simulink library "inp"  (R2021b)
settings: Solver=VariableStepAuto  StartTime=0.0  StopTime=10.0  RelTol=1e-3
undefined symbols (not defined in the file): C_TASK_5MS_S, FALSE, KINP_AcoreReadyToSlp_flg_ovrdflg, KINP_AcoreReadyToSlp_flg_ovrdval, KINP_AllowMovThd_OTA_enum_ovrdflg, KINP_AllowMovThd_OTA_enum_ovrdval, KINP_APSAngleTarget_Deg_ovrdflg, KINP_APSAngleTarget_Deg_ovrdval, KINP_APSDecReq_mps2_ovrdflg, KINP_APSDecReq_mps2_ovrdval, KINP_APSDecReqA_flg_ovrdflg, KINP_APSDecReqA_flg_ovrdval, KINP_APSDFLL_cm_ovrdflg, KINP_APSDFLL_cm_ovrdval, KINP_APSDFLR_cm_ovrdflg, KINP_APSDFLR_cm_ovrdval, KINP_APSDRLL_cm_ovrdflg, KINP_APSDRLL_cm_ovrdval, KINP_APSDRLR_cm_ovrdflg, KINP_APSDRLR_cm_ovrdval, KINP_APSExitCondition_enum_ovrdflg, KINP_APSExitCondition_enum_ovrdval, KINP_APSHWVer_enum_ovrdflg, KINP_APSHWVer_enum_ovrdval, KINP_APSProgressPCT_pct_ovrdflg, KINP_APSProgressPCT_pct_ovrdval, KINP_APSPwrReq_enum_ovrdflg, KINP_APSPwrReq_enum_ovrdval, KINP_APSReq_enum_ovrdflg, KINP_APSReq_enum_ovrdval, KINP_APSRQDisplay_enum_ovrdflg, KINP_APSRQDisplay_enum_ovrdval, KINP_APSRqEPASCtrl_flg_ovrdflg, KINP_APSRqEPASCtrl_flg_ovrdval, KINP_APSShiftPosnReq_enum_ovrdval, KINP_APSShiftPosnReq_enum_ovrflg, KINP_APSSpeedCMD_kph_ovrdval, KINP_APSSpeedCMD_kph_ovrflg, KINP_APSStaSystem_enum_ovrdflg, KINP_APSStaSystem_enum_ovrdval, KINP_APSSWVer_enum_ovrdflg, KINP_APSSWVer_enum_ovrdval, KINP_APSVMCReqA_flg_ovrdval, KINP_APSVMCReqA_flg_ovrflg, KINP_APSVRqEPASCtrl_flg_ovrdflg, KINP_APSVRqEPASCtrl_flg_ovrdval, KINP_AuxBattVolmV_mV_ovrdflg, KINP_AuxBattVolmV_mV_ovrdval, KINP_BTConnectSta_enum_ovrdflg, KINP_BTConnectSta_enum_ovrdval, KINP_CAASSta_enum_ovrdflg, KINP_CAASSta_enum_ovrdval, KINP_CAASVMCReqA_flg_ovrdval, KINP_CAASVMCReqA_flg_ovrflg, KINP_CAN1BusOff_flg_ovrdflg, KINP_CAN1BusOff_flg_ovrdval, KINP_CAN2BusOff_flg_ovrdflg, KINP_CAN2BusOff_flg_ovrdval, KINP_CAN3BusOff_flg_ovrdflg, KINP_CAN3BusOff_flg_ovrdval ... (+222)
libraries: FVT_lib x1035, hcu_lib x1
(part 21 of 33)

== system inp/INP/CAN3/SignalCheck/CCU2 ==
  BHAL_outputs : Inport
  inp_CanValid_bus : Inport  Port=2
  CCU2CSErr : FVT_lib/inp/can_signal_template  SystemSampleTime=-1  VariantActivationTime=update diagram  Latency=0  AutoFrameSizeCalculation=off
      link override defval: Value=KINP_CCU2CSErr_flg_defval
      link override ovrdflg: Value=KINP_CCU2CSErr_flg_ovrdflg
      link override ovrdval: Value=KINP_CCU2CSErr_flg_ovrdval
  CCU2RCErr : FVT_lib/inp/can_signal_template  SystemSampleTime=-1  VariantActivationTime=update diagram  Latency=0  AutoFrameSizeCalculation=off
      link override defval: Value=KINP_CCU2RCErr_flg_defval
      link override ovrdflg: Value=KINP_CCU2RCErr_flg_ovrdflg
      link override ovrdval: Value=KINP_CCU2RCErr_flg_ovrdval
  CSCCU2 : FVT_lib/inp/can_signal_template  SystemSampleTime=-1  VariantActivationTime=update diagram  Latency=0  AutoFrameSizeCalculation=off
      link override defval: Value=KINP_CSCCU2_enum_defval
      link override ovrdflg: Value=KINP_CSCCU2_enum_ovrdflg
      link override ovrdval: Value=KINP_CSCCU2_enum_ovrdval
  DCDCEnaSta : FVT_lib/inp/can_signal_template  SystemSampleTime=-1  VariantActivationTime=update diagram  Latency=0  AutoFrameSizeCalculation=off
      link override defval: Value=KINP_DCDCEnaSta_flg_defval
      link override ovrdflg: Value=KINP_DCDCEnaSta_flg_ovrdflg
      link override ovrdval: Value=KINP_DCDCEnaSta_flg_ovrdval
  DCDCFaultSta : FVT_lib/inp/can_signal_template  SystemSampleTime=-1  VariantActivationTime=update diagram  Latency=0  AutoFrameSizeCalculation=off
      link override defval: Value=KINP_DCDCFaultSta_enum_defval
      link override ovrdflg: Value=KINP_DCDCFaultSta_enum_ovrdflg
      link override ovrdval: Value=KINP_DCDCFaultSta_enum_ovrdval
  DCDCReady4Pre : FVT_lib/inp/can_signal_template  SystemSampleTime=-1  VariantActivationTime=update diagram  Latency=0  AutoFrameSizeCalculation=off
      link override defval: Value=KINP_DCDCReady4Pre_flg_defval
      link override ovrdflg: Value=KINP_DCDCReady4Pre_flg_ovrdflg
      link override ovrdval: Value=KINP_DCDCReady4Pre_flg_ovrdval
  DCDCTemp : FVT_lib/inp/can_signal_template  SystemSampleTime=-1  VariantActivationTime=update diagram  Latency=0  AutoFrameSizeCalculation=off
      link override defval: Value=KINP_DCDCTemp_C_defval
      link override ovrdflg: Value=KINP_DCDCTemp_C_ovrdflg
      link override ovrdval: Value=KINP_DCDCTemp_C_ovrdval
  OBCACCurLim : FVT_lib/inp/can_signal_template  SystemSampleTime=-1  VariantActivationTime=update diagram  Latency=0  AutoFrameSizeCalculation=off
      link override defval: Value=KINP_OBCACCurLim_enum_defval
      link override ovrdflg: Value=KINP_OBCACCurLim_enum_ovrdflg
      link override ovrdval: Value=KINP_OBCACCurLim_enum_ovrdval
  OBCACCurrInf : FVT_lib/inp/can_signal_template  SystemSampleTime=-1  VariantActivationTime=update diagram  Latency=0  AutoFrameSizeCalculation=off
      link override defval: Value=KINP_OBCACCurrInf_A_defval
      link override ovrdflg: Value=KINP_OBCACCurrInf_A_ovrdflg
      link override ovrdval: Value=KINP_OBCACCurrInf_A_ovrdval
  OBCACVoltInf : FVT_lib/inp/can_signal_template  SystemSampleTime=-1  VariantActivationTime=update diagram  Latency=0  AutoFrameSizeCalculation=off
      link override defval: Value=KINP_OBCACVoltInf_V_defval
      link override ovrdflg: Value=KINP_OBCACVoltInf_V_ovrdflg
      link override ovrdval: Value=KINP_OBCACVoltInf_V_ovrdval
  OBCEnaSta : FVT_lib/inp/can_signal_template  SystemSampleTime=-1  VariantActivationTime=update diagram  Latency=0  AutoFrameSizeCalculation=off
      link override defval: Value=KINP_OBCEnaSta_flg_defval
      link override ovrdflg: Value=KINP_OBCEnaSta_flg_ovrdflg
      link override ovrdval: Value=KINP_OBCEnaSta_flg_ovrdval
  OBCFaultSta : FVT_lib/inp/can_signal_template  SystemSampleTime=-1  VariantActivationTime=update diagram  Latency=0  AutoFrameSizeCalculation=off
      link override defval: Value=KINP_OBCFaultSta_enum_defval
      link override ovrdflg: Value=KINP_OBCFaultSta_enum_ovrdflg
      link override ovrdval: Value=KINP_OBCFaultSta_enum_ovrdval
  OBCPluginSta : FVT_lib/inp/can_signal_template  SystemSampleTime=-1  VariantActivationTime=update diagram  Latency=0  AutoFrameSizeCalculation=off
      link override defval: Value=KINP_OBCPluginSta_flg_defval
      link override ovrdflg: Value=KINP_OBCPluginSta_flg_ovrdflg
      link override ovrdval: Value=KINP_OBCPluginSta_flg_ovrdval
  OBCReady4Pre : FVT_lib/inp/can_signal_template  SystemSampleTime=-1  VariantActivationTime=update diagram  Latency=0  AutoFrameSizeCalculation=off
      link override defval: Value=KINP_OBCReady4Pre_flg_defval
      link override ovrdflg: Value=KINP_OBCReady4Pre_flg_ovrdflg
      link override ovrdval: Value=KINP_OBCReady4Pre_flg_ovrdval
  OBCTemp : FVT_lib/inp/can_signal_template  SystemSampleTime=-1  VariantActivationTime=update diagram  Latency=0  AutoFrameSizeCalculation=off
      link override defval: Value=KINP_OBCTemp_C_defval
      link override ovrdflg: Value=KINP_OBCTemp_C_ovrdflg
      link override ovrdval: Value=KINP_OBCTemp_C_ovrdval
  OBCV2LSta : FVT_lib/inp/can_signal_template  SystemSampleTime=-1  VariantActivationTime=update diagram  Latency=0  AutoFrameSizeCalculation=off
      link override defval: Value=KINP_OBCV2LSta_enum_defval
      link override ovrdflg: Value=KINP_OBCV2LSta_enum_ovrdflg
      link override ovrdval: Value=KINP_OBCV2LSta_enum_ovrdval
  RCCCU2 : FVT_lib/inp/can_signal_template  SystemSampleTime=-1  VariantActivationTime=update diagram  Latency=0  AutoFrameSizeCalculation=off
      link override defval: Value=KINP_RCCCU2_enum_defval
      link override ovrdflg: Value=KINP_RCCCU2_enum_ovrdflg
      link override ovrdval: Value=KINP_RCCCU2_enum_ovrdval
  Terminator_{1..17} (17 alike) : Terminator
  True_VHAL_CCU2CSErr_flg : Constant  Value=TRUE  OutDataTypeStr=boolean
  True_VHAL_CCU2RCErr_flg : Constant  Value=TRUE  OutDataTypeStr=boolean
  True_VHAL_CSCCU2_enum : Constant  Value=TRUE  OutDataTypeStr=boolean
  True_VHAL_DCDCEnaSta_flg : Constant  Value=TRUE  OutDataTypeStr=boolean
  True_VHAL_DCDCFaultSta_enum : Constant  Value=TRUE  OutDataTypeStr=boolean
  True_VHAL_DCDCReady4Pre_flg : Constant  Value=TRUE  OutDataTypeStr=boolean
  True_VHAL_DCDCTemp_C : Constant  Value=TRUE  OutDataTypeStr=boolean
  True_VHAL_OBCACCurLim_enum : Constant  Value=TRUE  OutDataTypeStr=boolean
  True_VHAL_OBCACCurrInf_A : Constant  Value=TRUE  OutDataTypeStr=boolean
  True_VHAL_OBCACVoltInf_V : Constant  Value=TRUE  OutDataTypeStr=boolean
  True_VHAL_OBCEnaSta_flg : Constant  Value=TRUE  OutDataTypeStr=boolean
  True_VHAL_OBCFaultSta_enum : Constant  Value=TRUE  OutDataTypeStr=boolean
  True_VHAL_OBCPluginSta_flg : Constant  Value=TRUE  OutDataTypeStr=boolean
  True_VHAL_OBCReady4Pre_flg : Constant  Value=TRUE  OutDataTypeStr=boolean
  True_VHAL_OBCTemp_C : Constant  Value=TRUE  OutDataTypeStr=boolean
  True_VHAL_OBCV2LSta_enum : Constant  Value=TRUE  OutDataTypeStr=boolean
  True_VHAL_RCCCU2_enum : Constant  Value=TRUE  OutDataTypeStr=boolean
  slr1_{1..17} (17 alike) : BusSelector  OutputSignals=VINP_CANMsgValidCCU2_flg
  slr_VHAL_CCU2CSErr_flg : BusSelector  OutputSignals=VHAL_CCU2CSErr_flg
  slr_VHAL_CCU2RCErr_flg : BusSelector  OutputSignals=VHAL_CCU2RCErr_flg
  slr_VHAL_CSCCU2_enum : BusSelector  OutputSignals=VHAL_CSCCU2_enum
  slr_VHAL_DCDCEnaSta_flg : BusSelector  OutputSignals=VHAL_DCDCEnaSta_flg
  slr_VHAL_DCDCFaultSta_enum : BusSelector  OutputSignals=VHAL_DCDCFaultSta_enum
  slr_VHAL_DCDCReady4Pre_flg : BusSelector  OutputSignals=VHAL_DCDCReady4Pre_flg
  slr_VHAL_DCDCTemp_C : BusSelector  OutputSignals=VHAL_DCDCTemp_C
  slr_VHAL_OBCACCurLim_enum : BusSelector  OutputSignals=VHAL_OBCACCurLim_enum
  slr_VHAL_OBCACCurrInf_A : BusSelector  OutputSignals=VHAL_OBCACCurrInf_A
  slr_VHAL_OBCACVoltInf_V : BusSelector  OutputSignals=VHAL_OBCACVoltInf_V
  slr_VHAL_OBCEnaSta_flg : BusSelector  OutputSignals=VHAL_OBCEnaSta_flg
  slr_VHAL_OBCFaultSta_enum : BusSelector  OutputSignals=VHAL_OBCFaultSta_enum
  slr_VHAL_OBCPluginSta_flg : BusSelector  OutputSignals=VHAL_OBCPluginSta_flg
  slr_VHAL_OBCReady4Pre_flg : BusSelector  OutputSignals=VHAL_OBCReady4Pre_flg
  slr_VHAL_OBCTemp_C : BusSelector  OutputSignals=VHAL_OBCTemp_C
  slr_VHAL_OBCV2LSta_enum : BusSelector  OutputSignals=VHAL_OBCV2LSta_enum
  slr_VHAL_RCCCU2_enum : BusSelector  OutputSignals=VHAL_RCCCU2_enum
  VINP_CCU2CSErr_flg : Outport
  VINP_CCU2RCErr_flg : Outport  Port=2
  VINP_CSCCU2_enum : Outport  Port=3
  VINP_DCDCEnaSta_flg : Outport  Port=4
  VINP_DCDCFaultSta_enum : Outport  Port=5
  VINP_DCDCReady4Pre_flg : Outport  Port=6
  VINP_DCDCTemp_C : Outport  Port=7
  VINP_OBCACCurrInf_A : Outport  Port=8
  VINP_OBCACVoltInf_V : Outport  Port=9
  VINP_OBCEnaSta_flg : Outport  Port=10
  VINP_OBCFaultSta_enum : Outport  Port=11
  VINP_OBCPluginSta_flg : Outport  Port=12
  VINP_OBCReady4Pre_flg : Outport  Port=13
  VINP_OBCTemp_C : Outport  Port=14
  VINP_OBCV2LSta_enum : Outport  Port=15
  VINP_OBCACCurLim_enum : Outport  Port=16
  VINP_RCCCU2_enum : Outport  Port=17
  wires:
  BHAL_outputs/1 -> [BHAL_outputs]
  inp_CanValid_bus/1 -> [inp_CanValid_bus]
  [BHAL_outputs] -> slr_VHAL_CCU2CSErr_flg/1
  slr_VHAL_CCU2CSErr_flg/1 -> CCU2CSErr/1  "<VHAL_CCU2CSErr_flg>"
  True_VHAL_CCU2CSErr_flg/1 -> CCU2CSErr/2
  [inp_CanValid_bus] -> slr1_1/1
  slr1_1/1 -> CCU2CSErr/3  "<VINP_CANMsgValidCCU2_flg>"
  CCU2CSErr/1 -> VINP_CCU2CSErr_flg/1  "VINP_CCU2CSErr_flg"
  CCU2CSErr/2 -> Terminator_1/1
  [BHAL_outputs] -> slr_VHAL_CCU2RCErr_flg/1
  slr_VHAL_CCU2RCErr_flg/1 -> CCU2RCErr/1  "<VHAL_CCU2RCErr_flg>"
  True_VHAL_CCU2RCErr_flg/1 -> CCU2RCErr/2
  [inp_CanValid_bus] -> slr1_2/1
  slr1_2/1 -> CCU2RCErr/3  "<VINP_CANMsgValidCCU2_flg>"
  CCU2RCErr/1 -> VINP_CCU2RCErr_flg/1  "VINP_CCU2RCErr_flg"
  CCU2RCErr/2 -> Terminator_2/1
  [BHAL_outputs] -> slr_VHAL_CSCCU2_enum/1
  slr_VHAL_CSCCU2_enum/1 -> CSCCU2/1  "<VHAL_CSCCU2_enum>"
  True_VHAL_CSCCU2_enum/1 -> CSCCU2/2
  [inp_CanValid_bus] -> slr1_3/1
  slr1_3/1 -> CSCCU2/3  "<VINP_CANMsgValidCCU2_flg>"
  CSCCU2/1 -> VINP_CSCCU2_enum/1  "VINP_CSCCU2_enum"
  CSCCU2/2 -> Terminator_3/1
  [BHAL_outputs] -> slr_VHAL_DCDCEnaSta_flg/1
  slr_VHAL_DCDCEnaSta_flg/1 -> DCDCEnaSta/1  "<VHAL_DCDCEnaSta_flg>"
  True_VHAL_DCDCEnaSta_flg/1 -> DCDCEnaSta/2
  [inp_CanValid_bus] -> slr1_4/1
  slr1_4/1 -> DCDCEnaSta/3  "<VINP_CANMsgValidCCU2_flg>"
  DCDCEnaSta/1 -> VINP_DCDCEnaSta_flg/1  "VINP_DCDCEnaSta_flg"
  DCDCEnaSta/2 -> Terminator_4/1
  [BHAL_outputs] -> slr_VHAL_DCDCFaultSta_enum/1
  slr_VHAL_DCDCFaultSta_enum/1 -> DCDCFaultSta/1  "<VHAL_DCDCFaultSta_enum>"
  True_VHAL_DCDCFaultSta_enum/1 -> DCDCFaultSta/2
  [inp_CanValid_bus] -> slr1_5/1
  slr1_5/1 -> DCDCFaultSta/3  "<VINP_CANMsgValidCCU2_flg>"
  DCDCFaultSta/1 -> VINP_DCDCFaultSta_enum/1  "VINP_DCDCFaultSta_enum"
  DCDCFaultSta/2 -> Terminator_5/1
  [BHAL_outputs] -> slr_VHAL_DCDCReady4Pre_flg/1
  slr_VHAL_DCDCReady4Pre_flg/1 -> DCDCReady4Pre/1  "<VHAL_DCDCReady4Pre_flg>"
  True_VHAL_DCDCReady4Pre_flg/1 -> DCDCReady4Pre/2
  [inp_CanValid_bus] -> slr1_6/1
  slr1_6/1 -> DCDCReady4Pre/3  "<VINP_CANMsgValidCCU2_flg>"
  DCDCReady4Pre/1 -> VINP_DCDCReady4Pre_flg/1  "VINP_DCDCReady4Pre_flg"
  DCDCReady4Pre/2 -> Terminator_6/1
  [BHAL_outputs] -> slr_VHAL_DCDCTemp_C/1
  slr_VHAL_DCDCTemp_C/1 -> DCDCTemp/1  "<VHAL_DCDCTemp_C>"
  True_VHAL_DCDCTemp_C/1 -> DCDCTemp/2
  [inp_CanValid_bus] -> slr1_7/1
  slr1_7/1 -> DCDCTemp/3  "<VINP_CANMsgValidCCU2_flg>"
  DCDCTemp/1 -> VINP_DCDCTemp_C/1  "VINP_DCDCTemp_C"
  DCDCTemp/2 -> Terminator_7/1
  [BHAL_outputs] -> slr_VHAL_OBCACCurrInf_A/1
  slr_VHAL_OBCACCurrInf_A/1 -> OBCACCurrInf/1  "<VHAL_OBCACCurrInf_A>"
  True_VHAL_OBCACCurrInf_A/1 -> OBCACCurrInf/2
  [inp_CanValid_bus] -> slr1_8/1
  slr1_8/1 -> OBCACCurrInf/3  "<VINP_CANMsgValidCCU2_flg>"
  OBCACCurrInf/1 -> VINP_OBCACCurrInf_A/1  "VINP_OBCACCurrInf_A"
  OBCACCurrInf/2 -> Terminator_8/1
  [BHAL_outputs] -> slr_VHAL_OBCACVoltInf_V/1
  slr_VHAL_OBCACVoltInf_V/1 -> OBCACVoltInf/1  "<VHAL_OBCACVoltInf_V>"
  True_VHAL_OBCACVoltInf_V/1 -> OBCACVoltInf/2
  [inp_CanValid_bus] -> slr1_9/1
  slr1_9/1 -> OBCACVoltInf/3  "<VINP_CANMsgValidCCU2_flg>"
  OBCACVoltInf/1 -> VINP_OBCACVoltInf_V/1  "VINP_OBCACVoltInf_V"
  OBCACVoltInf/2 -> Terminator_9/1
  [BHAL_outputs] -> slr_VHAL_OBCEnaSta_flg/1
  slr_VHAL_OBCEnaSta_flg/1 -> OBCEnaSta/1  "<VHAL_OBCEnaSta_flg>"
  True_VHAL_OBCEnaSta_flg/1 -> OBCEnaSta/2
  [inp_CanValid_bus] -> slr1_10/1
  slr1_10/1 -> OBCEnaSta/3  "<VINP_CANMsgValidCCU2_flg>"
  OBCEnaSta/1 -> VINP_OBCEnaSta_flg/1  "VINP_OBCEnaSta_flg"
  OBCEnaSta/2 -> Terminator_10/1
  [BHAL_outputs] -> slr_VHAL_OBCFaultSta_enum/1
  slr_VHAL_OBCFaultSta_enum/1 -> OBCFaultSta/1  "<VHAL_OBCFaultSta_enum>"
  True_VHAL_OBCFaultSta_enum/1 -> OBCFaultSta/2
  [inp_CanValid_bus] -> slr1_11/1
  slr1_11/1 -> OBCFaultSta/3  "<VINP_CANMsgValidCCU2_flg>"
  OBCFaultSta/1 -> VINP_OBCFaultSta_enum/1  "VINP_OBCFaultSta_enum"
  OBCFaultSta/2 -> Terminator_11/1
  [BHAL_outputs] -> slr_VHAL_OBCPluginSta_flg/1
  slr_VHAL_OBCPluginSta_flg/1 -> OBCPluginSta/1  "<VHAL_OBCPluginSta_flg>"
  True_VHAL_OBCPluginSta_flg/1 -> OBCPluginSta/2
  [inp_CanValid_bus] -> slr1_12/1
  slr1_12/1 -> OBCPluginSta/3  "<VINP_CANMsgValidCCU2_flg>"
  OBCPluginSta/1 -> VINP_OBCPluginSta_flg/1  "VINP_OBCPluginSta_flg"
  OBCPluginSta/2 -> Terminator_12/1
  [BHAL_outputs] -> slr_VHAL_OBCReady4Pre_flg/1
  slr_VHAL_OBCReady4Pre_flg/1 -> OBCReady4Pre/1  "<VHAL_OBCReady4Pre_flg>"
  True_VHAL_OBCReady4Pre_flg/1 -> OBCReady4Pre/2
  [inp_CanValid_bus] -> slr1_13/1
  slr1_13/1 -> OBCReady4Pre/3  "<VINP_CANMsgValidCCU2_flg>"
  OBCReady4Pre/1 -> VINP_OBCReady4Pre_flg/1  "VINP_OBCReady4Pre_flg"
  OBCReady4Pre/2 -> Terminator_13/1
  [BHAL_outputs] -> slr_VHAL_OBCTemp_C/1
  slr_VHAL_OBCTemp_C/1 -> OBCTemp/1  "<VHAL_OBCTemp_C>"
  True_VHAL_OBCTemp_C/1 -> OBCTemp/2
  [inp_CanValid_bus] -> slr1_14/1
  slr1_14/1 -> OBCTemp/3  "<VINP_CANMsgValidCCU2_flg>"
  OBCTemp/1 -> VINP_OBCTemp_C/1  "VINP_OBCTemp_C"
  OBCTemp/2 -> Terminator_14/1
  [BHAL_outputs] -> slr_VHAL_OBCV2LSta_enum/1
  slr_VHAL_OBCV2LSta_enum/1 -> OBCV2LSta/1  "<VHAL_OBCV2LSta_enum>"
  True_VHAL_OBCV2LSta_enum/1 -> OBCV2LSta/2
  [inp_CanValid_bus] -> slr1_15/1
  slr1_15/1 -> OBCV2LSta/3  "<VINP_CANMsgValidCCU2_flg>"
  OBCV2LSta/1 -> VINP_OBCV2LSta_enum/1  "VINP_OBCV2LSta_enum"
  OBCV2LSta/2 -> Terminator_15/1
  [BHAL_outputs] -> slr_VHAL_OBCACCurLim_enum/1
  slr_VHAL_OBCACCurLim_enum/1 -> OBCACCurLim/1  "<VHAL_OBCACCurLim_enum>"
  True_VHAL_OBCACCurLim_enum/1 -> OBCACCurLim/2
  [inp_CanValid_bus] -> slr1_16/1
  slr1_16/1 -> OBCACCurLim/3  "<VINP_CANMsgValidCCU2_flg>"
  OBCACCurLim/1 -> VINP_OBCACCurLim_enum/1  "VINP_OBCACCurLim_enum"
  OBCACCurLim/2 -> Terminator_16/1
  [BHAL_outputs] -> slr_VHAL_RCCCU2_enum/1
  slr_VHAL_RCCCU2_enum/1 -> RCCCU2/1  "<VHAL_RCCCU2_enum>"
  True_VHAL_RCCCU2_enum/1 -> RCCCU2/2
  [inp_CanValid_bus] -> slr1_17/1
  slr1_17/1 -> RCCCU2/3  "<VINP_CANMsgValidCCU2_flg>"
  RCCCU2/1 -> VINP_RCCCU2_enum/1  "VINP_RCCCU2_enum"
  RCCCU2/2 -> Terminator_17/1

== system inp/INP/CAN3/SignalCheck/EBM1 ==
  BHAL_outputs : Inport
  inp_CanValid_bus : Inport  Port=2
  EBMErrSta : FVT_lib/inp/can_signal_template  SystemSampleTime=-1  VariantActivationTime=update diagram  Latency=0  AutoFrameSizeCalculation=off
      link override defval: Value=KINP_EBMErrSta_enum_defval
      link override ovrdflg: Value=KINP_EBMErrSta_enum_ovrdflg
      link override ovrdval: Value=KINP_EBMErrSta_enum_ovrdval
  EBMRLampSta : FVT_lib/inp/can_signal_template  SystemSampleTime=-1  VariantActivationTime=update diagram  Latency=0  AutoFrameSizeCalculation=off
      link override defval: Value=KINP_EBMRLampSta_enum_defval
      link override ovrdflg: Value=KINP_EBMRLampSta_enum_ovrdflg
      link override ovrdval: Value=KINP_EBMRLampSta_enum_ovrdval
  Terminator_1 : Terminator
  Terminator_2 : Terminator
  True_VHAL_EBMErrSta_enum : Constant  Value=TRUE  OutDataTypeStr=boolean
  True_VHAL_EBMRLampSta_enum : Constant  Value=TRUE  OutDataTypeStr=boolean
  slr1_1 : BusSelector  OutputSignals=VINP_CANMsgValidEBM1_flg
  slr1_2 : BusSelector  OutputSignals=VINP_CANMsgValidEBM1_flg
  slr_VHAL_EBMErrSta_enum : BusSelector  OutputSignals=VHAL_EBMErrSta_enum
  slr_VHAL_EBMRLampSta_enum : BusSelector  OutputSignals=VHAL_EBMRLampSta_enum
  VINP_EBMErrSta_enum : Outport
  VINP_EBMRLampSta_enum : Outport  Port=2
  wires:
  BHAL_outputs/1 -> [BHAL_outputs]
  inp_CanValid_bus/1 -> [inp_CanValid_bus]
  [BHAL_outputs] -> slr_VHAL_EBMErrSta_enum/1
  slr_VHAL_EBMErrSta_enum/1 -> EBMErrSta/1  "<VHAL_EBMErrSta_enum>"
  True_VHAL_EBMErrSta_enum/1 -> EBMErrSta/2
  [inp_CanValid_bus] -> slr1_1/1
  slr1_1/1 -> EBMErrSta/3  "<VINP_CANMsgValidEBM1_flg>"
  EBMErrSta/1 -> VINP_EBMErrSta_enum/1  "VINP_EBMErrSta_enum"
  EBMErrSta/2 -> Terminator_1/1
  [BHAL_outputs] -> slr_VHAL_EBMRLampSta_enum/1
  slr_VHAL_EBMRLampSta_enum/1 -> EBMRLampSta/1  "<VHAL_EBMRLampSta_enum>"
  True_VHAL_EBMRLampSta_enum/1 -> EBMRLampSta/2
  [inp_CanValid_bus] -> slr1_2/1
  slr1_2/1 -> EBMRLampSta/3  "<VINP_CANMsgValidEBM1_flg>"
  EBMRLampSta/1 -> VINP_EBMRLampSta_enum/1  "VINP_EBMRLampSta_enum"
  EBMRLampSta/2 -> Terminator_2/1

== system inp/INP/CAN3/SignalCheck/MCU_B_F1 ==
  BHAL_outputs : Inport
  inp_CanValid_bus : Inport  Port=2
  FrActvDmpDisabSta : FVT_lib/inp/can_signal_template  SystemSampleTime=-1  VariantActivationTime=update diagram  Latency=0  AutoFrameSizeCalculation=off
      link override defval: Value=KINP_FrActvDmpDisabSta_flg_defval
      link override ovrdflg: Value=KINP_FrActvDmpDisabSta_flg_ovrdflg
      link override ovrdval: Value=KINP_FrActvDmpDisabSta_flg_ovrdval
  FrEDUDrtSta : FVT_lib/inp/can_signal_template  SystemSampleTime=-1  VariantActivationTime=update diagram  Latency=0  AutoFrameSizeCalculation=off
      link override defval: Value=KINP_FrEDUDrtSta_flg_defval
      link override ovrdflg: Value=KINP_FrEDUDrtSta_flg_ovrdflg
      link override ovrdval: Value=KINP_FrEDUDrtSta_flg_ovrdval
  FrEDUOpratingSta : FVT_lib/inp/can_signal_template  SystemSampleTime=-1  VariantActivationTime=update diagram  Latency=0  AutoFrameSizeCalculation=off
      link override defval: Value=KINP_FrEDUOpratingSta_flg_defval
      link override ovrdflg: Value=KINP_FrEDUOpratingSta_flg_ovrdflg
      link override ovrdval: Value=KINP_FrEDUOpratingSta_flg_ovrdval
  FrEDURealTMTq : FVT_lib/inp/can_signal_template  SystemSampleTime=-1  VariantActivationTime=update diagram  Latency=0  AutoFrameSizeCalculation=off
      link override defval: Value=KINP_FrEDURealTMTq_Nm_defval
      link override ovrdflg: Value=KINP_FrEDURealTMTq_Nm_ovrdflg
      link override ovrdval: Value=KINP_FrEDURealTMTq_Nm_ovrdval
  FrEDURotateDirction : FVT_lib/inp/can_signal_template  SystemSampleTime=-1  VariantActivationTime=update diagram  Latency=0  AutoFrameSizeCalculation=off
      link override defval: Value=KINP_FrEDURotateDirction_enum_defval
      link override ovrdflg: Value=KINP_FrEDURotateDirction_enum_ovrdflg
      link override ovrdval: Value=KINP_FrEDURotateDirction_enum_ovrdval
  FrEDUTqReqFbk : FVT_lib/inp/can_signal_template  SystemSampleTime=-1  VariantActivationTime=update diagram  Latency=0  AutoFrameSizeCalculation=off
      link override defval: Value=KINP_FrEDUTqReqFbk_Nm_defval
      link override ovrdflg: Value=KINP_FrEDUTqReqFbk_Nm_ovrdflg
      link override ovrdval: Value=KINP_FrEDUTqReqFbk_Nm_ovrdval
  FrMCU1Chksum : FVT_lib/inp/can_signal_template  SystemSampleTime=-1  VariantActivationTime=update diagram  Latency=0  AutoFrameSizeCalculation=off
      link override defval: Value=KINP_FrMCU1Chksum_enum_defval
      link override ovrdflg: Value=KINP_FrMCU1Chksum_enum_ovrdflg
      link override ovrdval: Value=KINP_FrMCU1Chksum_enum_ovrdval
  FrMCU1RolCnt : FVT_lib/inp/can_signal_template  SystemSampleTime=-1  VariantActivationTime=update diagram  Latency=0  AutoFrameSizeCalculation=off
      link override defval: Value=KINP_FrMCU1RolCnt_enum_defval
      link override ovrdflg: Value=KINP_FrMCU1RolCnt_enum_ovrdflg
      link override ovrdval: Value=KINP_FrMCU1RolCnt_enum_ovrdval
  FrMCUBAT : FVT_lib/inp/can_signal_template  SystemSampleTime=-1  VariantActivationTime=update diagram  Latency=0  AutoFrameSizeCalculation=off
      link override defval: Value=KINP_FrMCUBAT_V_defval
      link override ovrdflg: Value=KINP_FrMCUBAT_V_ovrdflg
      link override ovrdval: Value=KINP_FrMCUBAT_V_ovrdval
  FrMCUDCBusCurr : FVT_lib/inp/can_signal_template  SystemSampleTime=-1  VariantActivationTime=update diagram  Latency=0  AutoFrameSizeCalculation=off
      link override defval: Value=KINP_FrMCUDCBusCurr_A_defval
      link override ovrdflg: Value=KINP_FrMCUDCBusCurr_A_ovrdflg
      link override ovrdval: Value=KINP_FrMCUDCBusCurr_A_ovrdval
  FrMCUDCBusVolt : FVT_lib/inp/can_signal_template  SystemSampleTime=-1  VariantActivationTime=update diagram  Latency=0  AutoFrameSizeCalculation=off
      link override defval: Value=KINP_FrMCUDCBusVolt_V_defval
      link override ovrdflg: Value=KINP_FrMCUDCBusVolt_V_ovrdflg
      link override ovrdval: Value=KINP_FrMCUDCBusVolt_V_ovrdval
  FrMCUDischrgSta : FVT_lib/inp/can_signal_template  SystemSampleTime=-1  VariantActivationTime=update diagram  Latency=0  AutoFrameSizeCalculation=off
      link override defval: Value=KINP_FrMCUDischrgSta_flg_defval
      link override ovrdflg: Value=KINP_FrMCUDischrgSta_flg_ovrdflg
      link override ovrdval: Value=KINP_FrMCUDischrgSta_flg_ovrdval
  FrMCUEnaSta : FVT_lib/inp/can_signal_template  SystemSampleTime=-1  VariantActivationTime=update diagram  Latency=0  AutoFrameSizeCalculation=off
      link override defval: Value=KINP_FrMCUEnaSta_flg_defval
      link override ovrdflg: Value=KINP_FrMCUEnaSta_flg_ovrdflg
      link override ovrdval: Value=KINP_FrMCUEnaSta_flg_ovrdval
  FrMCUErr : FVT_lib/inp/can_signal_template  SystemSampleTime=-1  VariantActivationTime=update diagram  Latency=0  AutoFrameSizeCalculation=off
      link override defval: Value=KINP_FrMCUErr_enum_defval
      link override ovrdflg: Value=KINP_FrMCUErr_enum_ovrdflg
      link override ovrdval: Value=KINP_FrMCUErr_enum_ovrdval
  FrMCUIGNsta : FVT_lib/inp/can_signal_template  SystemSampleTime=-1  VariantActivationTime=update diagram  Latency=0  AutoFrameSizeCalculation=off
      link override defval: Value=KINP_FrMCUIGNsta_flg_defval
      link override ovrdflg: Value=KINP_FrMCUIGNsta_flg_ovrdflg
      link override ovrdval: Value=KINP_FrMCUIGNsta_flg_ovrdval
  FrMCUReady : FVT_lib/inp/can_signal_template  SystemSampleTime=-1  VariantActivationTime=update diagram  Latency=0  AutoFrameSizeCalculation=off
      link override defval: Value=KINP_FrMCUReady_flg_defval
      link override ovrdflg: Value=KINP_FrMCUReady_flg_ovrdflg
      link override ovrdval: Value=KINP_FrMCUReady_flg_ovrdval
  FrMCUReady4Pre : FVT_lib/inp/can_signal_template  SystemSampleTime=-1  VariantActivationTime=update diagram  Latency=0  AutoFrameSizeCalculation=off
      link override defval: Value=KINP_FrMCUReady4Pre_flg_defval
      link override ovrdflg: Value=KINP_FrMCUReady4Pre_flg_ovrdflg
      link override ovrdval: Value=KINP_FrMCUReady4Pre_flg_ovrdval
  FrMCUSysSta : FVT_lib/inp/can_signal_template  SystemSampleTime=-1  VariantActivationTime=update diagram  Latency=0  AutoFrameSizeCalculation=off
      link override defval: Value=KINP_FrMCUSysSta_enum_defval
      link override ovrdflg: Value=KINP_FrMCUSysSta_enum_ovrdflg
      link override ovrdval: Value=KINP_FrMCUSysSta_enum_ovrdval
  FrMCUTemp : FVT_lib/inp/can_signal_template  SystemSampleTime=-1  VariantActivationTime=update diagram  Latency=0  AutoFrameSizeCalculation=off
      link override defval: Value=KINP_FrMCUTemp_C_defval
      link override ovrdflg: Value=KINP_FrMCUTemp_C_ovrdflg
      link override ovrdval: Value=KINP_FrMCUTemp_C_ovrdval
  FrMotorAvailTq : FVT_lib/inp/can_signal_template  SystemSampleTime=-1  VariantActivationTime=update diagram  Latency=0  AutoFrameSizeCalculation=off
      link override defval: Value=KINP_FrMotorAvailTq_Nm_defval
      link override ovrdflg: Value=KINP_FrMotorAvailTq_Nm_ovrdflg
      link override ovrdval: Value=KINP_FrMotorAvailTq_Nm_ovrdval
  FrRegenAvailTq : FVT_lib/inp/can_signal_template  SystemSampleTime=-1  VariantActivationTime=update diagram  Latency=0  AutoFrameSizeCalculation=off
      link override defval: Value=KINP_FrRegenAvailTq_Nm_defval
      link override ovrdflg: Value=KINP_FrRegenAvailTq_Nm_ovrdflg
      link override ovrdval: Value=KINP_FrRegenAvailTq_Nm_ovrdval
  FrTMSpd : FVT_lib/inp/can_signal_template  SystemSampleTime=-1  VariantActivationTime=update diagram  Latency=0  AutoFrameSizeCalculation=off
      link override defval: Value=KINP_FrTMSpd_rpm_defval
      link override ovrdflg: Value=KINP_FrTMSpd_rpm_ovrdflg
      link override ovrdval: Value=KINP_FrTMSpd_rpm_ovrdval
  FrTMTemp : FVT_lib/inp/can_signal_template  SystemSampleTime=-1  VariantActivationTime=update diagram  Latency=0  AutoFrameSizeCalculation=off
      link override defval: Value=KINP_FrTMTemp_C_defval
      link override ovrdflg: Value=KINP_FrTMTemp_C_ovrdflg
      link override ovrdval: Value=KINP_FrTMTemp_C_ovrdval
  FrTMid : FVT_lib/inp/can_signal_template  SystemSampleTime=-1  VariantActivationTime=update diagram  Latency=0  AutoFrameSizeCalculation=off
      link override defval: Value=KINP_FrTMid_A_defval
      link override ovrdflg: Value=KINP_FrTMid_A_ovrdflg
      link override ovrdval: Value=KINP_FrTMid_A_ovrdval
  FrTMiq : FVT_lib/inp/can_signal_template  SystemSampleTime=-1  VariantActivationTime=update diagram  Latency=0  AutoFrameSizeCalculation=off
      link override defval: Value=KINP_FrTMiq_A_defval
      link override ovrdflg: Value=KINP_FrTMiq_A_ovrdflg
      link override ovrdval: Value=KINP_FrTMiq_A_ovrdval
  MCUBF1CSErr : FVT_lib/inp/can_signal_template  SystemSampleTime=-1  VariantActivationTime=update diagram  Latency=0  AutoFrameSizeCalculation=off
      link override defval: Value=KINP_MCUBF1CSErr_flg_defval
      link override ovrdflg: Value=KINP_MCUBF1CSErr_flg_ovrdflg
      link override ovrdval: Value=KINP_MCUBF1CSErr_flg_ovrdval
  MCUBF1RCErr : FVT_lib/inp/can_signal_template  SystemSampleTime=-1  VariantActivationTime=update diagram  Latency=0  AutoFrameSizeCalculation=off
      link override defval: Value=KINP_MCUBF1RCErr_flg_defval
      link override ovrdflg: Value=KINP_MCUBF1RCErr_flg_ovrdflg
      link override ovrdval: Value=KINP_MCUBF1RCErr_flg_ovrdval
  MCUBFRealPwrKwSta : FVT_lib/inp/can_signal_template  SystemSampleTime=-1  VariantActivationTime=update diagram  Latency=0  AutoFrameSizeCalculation=off
      link override defval: Value=KINP_MCUBFRealPwrKwSta_kW_defval
      link override ovrdflg: Value=KINP_MCUBFRealPwrKwSta_kW_ovrdflg
      link override ovrdval: Value=KINP_MCUBFRealPwrKwSta_kW_ovrdval
  MCUWarnF : FVT_lib/inp/can_signal_template  SystemSampleTime=-1  VariantActivationTime=update diagram  Latency=0  AutoFrameSizeCalculation=off
      link override defval: Value=KINP_MCUWarnF_enum_defval
      link override ovrdflg: Value=KINP_MCUWarnF_enum_ovrdflg
      link override ovrdval: Value=KINP_MCUWarnF_enum_ovrdval
  Terminator_{1..29} (29 alike) : Terminator
  True_VHAL_FrActvDmpDisabSta_flg : Constant  Value=TRUE  OutDataTypeStr=boolean
  True_VHAL_FrEDUDrtSta_flg : Constant  Value=TRUE  OutDataTypeStr=boolean
  True_VHAL_FrEDUOpratingSta_flg : Constant  Value=TRUE  OutDataTypeStr=boolean
  True_VHAL_FrEDURealTMTq_Nm : Constant  Value=TRUE  OutDataTypeStr=boolean
  True_VHAL_FrEDURotateDirction_enum : Constant  Value=TRUE  OutDataTypeStr=boolean
  True_VHAL_FrEDUTqReqFbk_Nm : Constant  Value=TRUE  OutDataTypeStr=boolean
  True_VHAL_FrMCU1Chksum_enum : Constant  Value=TRUE  OutDataTypeStr=boolean
  True_VHAL_FrMCU1RolCnt_enum : Constant  Value=TRUE  OutDataTypeStr=boolean
  True_VHAL_FrMCUBAT_V : Constant  Value=TRUE  OutDataTypeStr=boolean
  True_VHAL_FrMCUDCBusCurr_A : Constant  Value=TRUE  OutDataTypeStr=boolean
  True_VHAL_FrMCUDCBusVolt_V : Constant  Value=TRUE  OutDataTypeStr=boolean
  True_VHAL_FrMCUDischrgSta_flg : Constant  Value=TRUE  OutDataTypeStr=boolean
  True_VHAL_FrMCUEnaSta_flg : Constant  Value=TRUE  OutDataTypeStr=boolean
  True_VHAL_FrMCUErr_enum : Constant  Value=TRUE  OutDataTypeStr=boolean
  True_VHAL_FrMCUIGNsta_flg : Constant  Value=TRUE  OutDataTypeStr=boolean
  True_VHAL_FrMCUReady4Pre_flg : Constant  Value=TRUE  OutDataTypeStr=boolean
  True_VHAL_FrMCUReady_flg : Constant  Value=TRUE  OutDataTypeStr=boolean
  True_VHAL_FrMCUSysSta_enum : Constant  Value=TRUE  OutDataTypeStr=boolean
  True_VHAL_FrMCUTemp_C : Constant  Value=TRUE  OutDataTypeStr=boolean
  True_VHAL_FrMotorAvailTq_Nm : Constant  Value=TRUE  OutDataTypeStr=boolean
  True_VHAL_FrRegenAvailTq_Nm : Constant  Value=TRUE  OutDataTypeStr=boolean
  True_VHAL_FrTMSpd_rpm : Constant  Value=TRUE  OutDataTypeStr=boolean
  True_VHAL_FrTMTemp_C : Constant  Value=TRUE  OutDataTypeStr=boolean
  True_VHAL_FrTMid_A : Constant  Value=TRUE  OutDataTypeStr=boolean
  True_VHAL_FrTMiq_A : Constant  Value=TRUE  OutDataTypeStr=boolean
  True_VHAL_MCUBF1CSErr_flg : Constant  Value=TRUE  OutDataTypeStr=boolean
  True_VHAL_MCUBF1RCErr_flg : Constant  Value=TRUE  OutDataTypeStr=boolean
  True_VHAL_MCUBFRealPwrKwSta_kW : Constant  Value=TRUE  OutDataTypeStr=boolean
  True_VHAL_MCUWarnF_enum : Constant  Value=TRUE  OutDataTypeStr=boolean
  slr1_{1..29} (29 alike) : BusSelector  OutputSignals=VINP_CANMsgValidMCUBF1_flg
  slr_VHAL_FrActvDmpDisabSta_flg : BusSelector  OutputSignals=VHAL_FrActvDmpDisabSta_flg
  slr_VHAL_FrEDUDrtSta_flg : BusSelector  OutputSignals=VHAL_FrEDUDrtSta_flg
  slr_VHAL_FrEDUOpratingSta_flg : BusSelector  OutputSignals=VHAL_FrEDUOpratingSta_flg
  slr_VHAL_FrEDURealTMTq_Nm : BusSelector  OutputSignals=VHAL_FrEDURealTMTq_Nm
  slr_VHAL_FrEDURotateDirction_enum : BusSelector  OutputSignals=VHAL_FrEDURotateDirction_enum
  slr_VHAL_FrEDUTqReqFbk_Nm : BusSelector  OutputSignals=VHAL_FrEDUTqReqFbk_Nm
  slr_VHAL_FrMCU1Chksum_enum : BusSelector  OutputSignals=VHAL_FrMCU1Chksum_enum
  slr_VHAL_FrMCU1RolCnt_enum : BusSelector  OutputSignals=VHAL_FrMCU1RolCnt_enum
  slr_VHAL_FrMCUBAT_V : BusSelector  OutputSignals=VHAL_FrMCUBAT_V
  slr_VHAL_FrMCUDCBusCurr_A : BusSelector  OutputSignals=VHAL_FrMCUDCBusCurr_A
  slr_VHAL_FrMCUDCBusVolt_V : BusSelector  OutputSignals=VHAL_FrMCUDCBusVolt_V
  slr_VHAL_FrMCUDischrgSta_flg : BusSelector  OutputSignals=VHAL_FrMCUDischrgSta_flg
  slr_VHAL_FrMCUEnaSta_flg : BusSelector  OutputSignals=VHAL_FrMCUEnaSta_flg
  slr_VHAL_FrMCUErr_enum : BusSelector  OutputSignals=VHAL_FrMCUErr_enum
  slr_VHAL_FrMCUIGNsta_flg : BusSelector  OutputSignals=VHAL_FrMCUIGNsta_flg
  slr_VHAL_FrMCUReady4Pre_flg : BusSelector  OutputSignals=VHAL_FrMCUReady4Pre_flg
  slr_VHAL_FrMCUReady_flg : BusSelector  OutputSignals=VHAL_FrMCUReady_flg
  slr_VHAL_FrMCUSysSta_enum : BusSelector  OutputSignals=VHAL_FrMCUSysSta_enum
  slr_VHAL_FrMCUTemp_C : BusSelector  OutputSignals=VHAL_FrMCUTemp_C
  slr_VHAL_FrMotorAvailTq_Nm : BusSelector  OutputSignals=VHAL_FrMotorAvailTq_Nm
  slr_VHAL_FrRegenAvailTq_Nm : BusSelector  OutputSignals=VHAL_FrRegenAvailTq_Nm
  slr_VHAL_FrTMSpd_rpm : BusSelector  OutputSignals=VHAL_FrTMSpd_rpm
  slr_VHAL_FrTMTemp_C : BusSelector  OutputSignals=VHAL_FrTMTemp_C
  slr_VHAL_FrTMid_A : BusSelector  OutputSignals=VHAL_FrTMid_A
  slr_VHAL_FrTMiq_A : BusSelector  OutputSignals=VHAL_FrTMiq_A
  slr_VHAL_MCUBF1CSErr_flg : BusSelector  OutputSignals=VHAL_MCUBF1CSErr_flg
  slr_VHAL_MCUBF1RCErr_flg : BusSelector  OutputSignals=VHAL_MCUBF1RCErr_flg
  slr_VHAL_MCUBFRealPwrKwSta_kW : BusSelector  OutputSignals=VHAL_MCUBFRealPwrKwSta_kW
  slr_VHAL_MCUWarnF_enum : BusSelector  OutputSignals=VHAL_MCUWarnF_enum
  VINP_MCUBF1CSErr_flg : Outport
  VINP_MCUBF1RCErr_flg : Outport  Port=2
  VINP_FrActvDmpDisabSta_flg : Outport  Port=3
  VINP_FrEDUDrtSta_flg : Outport  Port=4
  VINP_FrEDUOpratingSta_flg : Outport  Port=5
  VINP_FrEDURealTMTq_Nm : Outport  Port=6
  VINP_FrEDURotateDirction_enum : Outport  Port=7
  VINP_FrEDUTqReqFbk_Nm : Outport  Port=8
  VINP_FrMCU1Chksum_enum : Outport  Port=9
  VINP_FrMCU1RolCnt_enum : Outport  Port=10
  VINP_FrMCUBAT_V : Outport  Port=11
  VINP_FrMCUDCBusCurr_A : Outport  Port=12
  VINP_FrMCUDCBusVolt_V : Outport  Port=13
  VINP_FrMCUDischrgSta_flg : Outport  Port=14
  VINP_FrMCUEnaSta_flg : Outport  Port=15
  VINP_FrMCUErr_enum : Outport  Port=16
  VINP_FrMCUIGNsta_flg : Outport  Port=17
  VINP_FrMCUReady_flg : Outport  Port=18
  VINP_FrMCUReady4Pre_flg : Outport  Port=19
  VINP_FrMCUSysSta_enum : Outport  Port=20
  VINP_FrMCUTemp_C : Outport  Port=21
  VINP_FrMotorAvailTq_Nm : Outport  Port=22
  VINP_FrRegenAvailTq_Nm : Outport  Port=23
  VINP_FrTMSpd_rpm : Outport  Port=24
  VINP_FrTMTemp_C : Outport  Port=25
  VINP_FrTMid_A : Outport  Port=26
  VINP_FrTMiq_A : Outport  Port=27
  VINP_MCUWarnF_enum : Outport  Port=28
  VINP_MCUBFRealPwrKwSta_kW : Outport  Port=29
  wires:
  BHAL_outputs/1 -> [BHAL_outputs]
  inp_CanValid_bus/1 -> [inp_CanValid_bus]
  [BHAL_outputs] -> slr_VHAL_MCUBF1CSErr_flg/1
  slr_VHAL_MCUBF1CSErr_flg/1 -> MCUBF1CSErr/1  "<VHAL_MCUBF1CSErr_flg>"
  True_VHAL_MCUBF1CSErr_flg/1 -> MCUBF1CSErr/2
  [inp_CanValid_bus] -> slr1_1/1
  slr1_1/1 -> MCUBF1CSErr/3  "<VINP_CANMsgValidMCUBF1_flg>"
  MCUBF1CSErr/1 -> VINP_MCUBF1CSErr_flg/1  "VINP_MCUBF1CSErr_flg"
  MCUBF1CSErr/2 -> Terminator_1/1
  [BHAL_outputs] -> slr_VHAL_MCUBF1RCErr_flg/1
  slr_VHAL_MCUBF1RCErr_flg/1 -> MCUBF1RCErr/1  "<VHAL_MCUBF1RCErr_flg>"
  True_VHAL_MCUBF1RCErr_flg/1 -> MCUBF1RCErr/2
  [inp_CanValid_bus] -> slr1_2/1
  slr1_2/1 -> MCUBF1RCErr/3  "<VINP_CANMsgValidMCUBF1_flg>"
  MCUBF1RCErr/1 -> VINP_MCUBF1RCErr_flg/1  "VINP_MCUBF1RCErr_flg"
  MCUBF1RCErr/2 -> Terminator_2/1
  [BHAL_outputs] -> slr_VHAL_FrActvDmpDisabSta_flg/1
  slr_VHAL_FrActvDmpDisabSta_flg/1 -> FrActvDmpDisabSta/1  "<VHAL_FrActvDmpDisabSta_flg>"
  True_VHAL_FrActvDmpDisabSta_flg/1 -> FrActvDmpDisabSta/2
  [inp_CanValid_bus] -> slr1_3/1
  slr1_3/1 -> FrActvDmpDisabSta/3  "<VINP_CANMsgValidMCUBF1_flg>"
  FrActvDmpDisabSta/1 -> VINP_FrActvDmpDisabSta_flg/1  "VINP_FrActvDmpDisabSta_flg"
  FrActvDmpDisabSta/2 -> Terminator_3/1
  [BHAL_outputs] -> slr_VHAL_FrEDUDrtSta_flg/1
  slr_VHAL_FrEDUDrtSta_flg/1 -> FrEDUDrtSta/1  "<VHAL_FrEDUDrtSta_flg>"
  True_VHAL_FrEDUDrtSta_flg/1 -> FrEDUDrtSta/2
  [inp_CanValid_bus] -> slr1_4/1
  slr1_4/1 -> FrEDUDrtSta/3  "<VINP_CANMsgValidMCUBF1_flg>"
  FrEDUDrtSta/1 -> VINP_FrEDUDrtSta_flg/1  "VINP_FrEDUDrtSta_flg"
  FrEDUDrtSta/2 -> Terminator_4/1
  [BHAL_outputs] -> slr_VHAL_FrEDUOpratingSta_flg/1
  slr_VHAL_FrEDUOpratingSta_flg/1 -> FrEDUOpratingSta/1  "<VHAL_FrEDUOpratingSta_flg>"
  True_VHAL_FrEDUOpratingSta_flg/1 -> FrEDUOpratingSta/2
  [inp_CanValid_bus] -> slr1_5/1
  slr1_5/1 -> FrEDUOpratingSta/3  "<VINP_CANMsgValidMCUBF1_flg>"
  FrEDUOpratingSta/1 -> VINP_FrEDUOpratingSta_flg/1  "VINP_FrEDUOpratingSta_flg"
  FrEDUOpratingSta/2 -> Terminator_5/1
  [BHAL_outputs] -> slr_VHAL_FrEDURealTMTq_Nm/1
  slr_VHAL_FrEDURealTMTq_Nm/1 -> FrEDURealTMTq/1  "<VHAL_FrEDURealTMTq_Nm>"
  True_VHAL_FrEDURealTMTq_Nm/1 -> FrEDURealTMTq/2
  [inp_CanValid_bus] -> slr1_6/1
  slr1_6/1 -> FrEDURealTMTq/3  "<VINP_CANMsgValidMCUBF1_flg>"
  FrEDURealTMTq/1 -> VINP_FrEDURealTMTq_Nm/1  "VINP_FrEDURealTMTq_Nm"
  FrEDURealTMTq/2 -> Terminator_6/1
  [BHAL_outputs] -> slr_VHAL_FrEDURotateDirction_enum/1
  slr_VHAL_FrEDURotateDirction_enum/1 -> FrEDURotateDirction/1  "<VHAL_FrEDURotateDirction_enum>"
  True_VHAL_FrEDURotateDirction_enum/1 -> FrEDURotateDirction/2
  [inp_CanValid_bus] -> slr1_7/1
  slr1_7/1 -> FrEDURotateDirction/3  "<VINP_CANMsgValidMCUBF1_flg>"
  FrEDURotateDirction/1 -> VINP_FrEDURotateDirction_enum/1  "VINP_FrEDURotateDirction_enum"
  FrEDURotateDirction/2 -> Terminator_7/1
  [BHAL_outputs] -> slr_VHAL_FrEDUTqReqFbk_Nm/1
  slr_VHAL_FrEDUTqReqFbk_Nm/1 -> FrEDUTqReqFbk/1  "<VHAL_FrEDUTqReqFbk_Nm>"
  True_VHAL_FrEDUTqReqFbk_Nm/1 -> FrEDUTqReqFbk/2
  [inp_CanValid_bus] -> slr1_8/1
  slr1_8/1 -> FrEDUTqReqFbk/3  "<VINP_CANMsgValidMCUBF1_flg>"
  FrEDUTqReqFbk/1 -> VINP_FrEDUTqReqFbk_Nm/1  "VINP_FrEDUTqReqFbk_Nm"
  FrEDUTqReqFbk/2 -> Terminator_8/1
  [BHAL_outputs] -> slr_VHAL_FrMCU1Chksum_enum/1
  slr_VHAL_FrMCU1Chksum_enum/1 -> FrMCU1Chksum/1  "<VHAL_FrMCU1Chksum_enum>"
  True_VHAL_FrMCU1Chksum_enum/1 -> FrMCU1Chksum/2
  [inp_CanValid_bus] -> slr1_9/1
  slr1_9/1 -> FrMCU1Chksum/3  "<VINP_CANMsgValidMCUBF1_flg>"
  FrMCU1Chksum/1 -> VINP_FrMCU1Chksum_enum/1  "VINP_FrMCU1Chksum_enum"
  FrMCU1Chksum/2 -> Terminator_9/1
  [BHAL_outputs] -> slr_VHAL_FrMCU1RolCnt_enum/1
  slr_VHAL_FrMCU1RolCnt_enum/1 -> FrMCU1RolCnt/1  "<VHAL_FrMCU1RolCnt_enum>"
  True_VHAL_FrMCU1RolCnt_enum/1 -> FrMCU1RolCnt/2
  [inp_CanValid_bus] -> slr1_10/1
  slr1_10/1 -> FrMCU1RolCnt/3  "<VINP_CANMsgValidMCUBF1_flg>"
  FrMCU1RolCnt/1 -> VINP_FrMCU1RolCnt_enum/1  "VINP_FrMCU1RolCnt_enum"
  FrMCU1RolCnt/2 -> Terminator_10/1
  [BHAL_outputs] -> slr_VHAL_FrMCUBAT_V/1
  slr_VHAL_FrMCUBAT_V/1 -> FrMCUBAT/1  "<VHAL_FrMCUBAT_V>"
  True_VHAL_FrMCUBAT_V/1 -> FrMCUBAT/2
  [inp_CanValid_bus] -> slr1_11/1
  slr1_11/1 -> FrMCUBAT/3  "<VINP_CANMsgValidMCUBF1_flg>"
  FrMCUBAT/1 -> VINP_FrMCUBAT_V/1  "VINP_FrMCUBAT_V"
  FrMCUBAT/2 -> Terminator_11/1
  [BHAL_outputs] -> slr_VHAL_FrMCUDCBusCurr_A/1
  slr_VHAL_FrMCUDCBusCurr_A/1 -> FrMCUDCBusCurr/1  "<VHAL_FrMCUDCBusCurr_A>"
  True_VHAL_FrMCUDCBusCurr_A/1 -> FrMCUDCBusCurr/2
  [inp_CanValid_bus] -> slr1_12/1
  slr1_12/1 -> FrMCUDCBusCurr/3  "<VINP_CANMsgValidMCUBF1_flg>"
  FrMCUDCBusCurr/1 -> VINP_FrMCUDCBusCurr_A/1  "VINP_FrMCUDCBusCurr_A"
  FrMCUDCBusCurr/2 -> Terminator_12/1
  [BHAL_outputs] -> slr_VHAL_FrMCUDCBusVolt_V/1
  slr_VHAL_FrMCUDCBusVolt_V/1 -> FrMCUDCBusVolt/1  "<VHAL_FrMCUDCBusVolt_V>"
  True_VHAL_FrMCUDCBusVolt_V/1 -> FrMCUDCBusVolt/2
  [inp_CanValid_bus] -> slr1_13/1
  slr1_13/1 -> FrMCUDCBusVolt/3  "<VINP_CANMsgValidMCUBF1_flg>"
  FrMCUDCBusVolt/1 -> VINP_FrMCUDCBusVolt_V/1  "VINP_FrMCUDCBusVolt_V"
  FrMCUDCBusVolt/2 -> Terminator_13/1
  [BHAL_outputs] -> slr_VHAL_FrMCUDischrgSta_flg/1
  slr_VHAL_FrMCUDischrgSta_flg/1 -> FrMCUDischrgSta/1  "<VHAL_FrMCUDischrgSta_flg>"
  True_VHAL_FrMCUDischrgSta_flg/1 -> FrMCUDischrgSta/2
  [inp_CanValid_bus] -> slr1_14/1
  slr1_14/1 -> FrMCUDischrgSta/3  "<VINP_CANMsgValidMCUBF1_flg>"
  FrMCUDischrgSta/1 -> VINP_FrMCUDischrgSta_flg/1  "VINP_FrMCUDischrgSta_flg"
  FrMCUDischrgSta/2 -> Terminator_14/1
  [BHAL_outputs] -> slr_VHAL_FrMCUEnaSta_flg/1
  slr_VHAL_FrMCUEnaSta_flg/1 -> FrMCUEnaSta/1  "<VHAL_FrMCUEnaSta_flg>"
  True_VHAL_FrMCUEnaSta_flg/1 -> FrMCUEnaSta/2
  [inp_CanValid_bus] -> slr1_15/1
  slr1_15/1 -> FrMCUEnaSta/3  "<VINP_CANMsgValidMCUBF1_flg>"
  FrMCUEnaSta/1 -> VINP_FrMCUEnaSta_flg/1  "VINP_FrMCUEnaSta_flg"
  FrMCUEnaSta/2 -> Terminator_15/1
  [BHAL_outputs] -> slr_VHAL_FrMCUErr_enum/1
  slr_VHAL_FrMCUErr_enum/1 -> FrMCUErr/1  "<VHAL_FrMCUErr_enum>"
  True_VHAL_FrMCUErr_enum/1 -> FrMCUErr/2
  [inp_CanValid_bus] -> slr1_16/1
  slr1_16/1 -> FrMCUErr/3  "<VINP_CANMsgValidMCUBF1_flg>"
  FrMCUErr/1 -> VINP_FrMCUErr_enum/1  "VINP_FrMCUErr_enum"
  FrMCUErr/2 -> Terminator_16/1
  [BHAL_outputs] -> slr_VHAL_FrMCUIGNsta_flg/1
  slr_VHAL_FrMCUIGNsta_flg/1 -> FrMCUIGNsta/1  "<VHAL_FrMCUIGNsta_flg>"
  True_VHAL_FrMCUIGNsta_flg/1 -> FrMCUIGNsta/2
  [inp_CanValid_bus] -> slr1_17/1
  slr1_17/1 -> FrMCUIGNsta/3  "<VINP_CANMsgValidMCUBF1_flg>"
  FrMCUIGNsta/1 -> VINP_FrMCUIGNsta_flg/1  "VINP_FrMCUIGNsta_flg"
  FrMCUIGNsta/2 -> Terminator_17/1
  [BHAL_outputs] -> slr_VHAL_FrMCUReady_flg/1
  slr_VHAL_FrMCUReady_flg/1 -> FrMCUReady/1  "<VHAL_FrMCUReady_flg>"
  True_VHAL_FrMCUReady_flg/1 -> FrMCUReady/2
  [inp_CanValid_bus] -> slr1_18/1
  slr1_18/1 -> FrMCUReady/3  "<VINP_CANMsgValidMCUBF1_flg>"
  FrMCUReady/1 -> VINP_FrMCUReady_flg/1  "VINP_FrMCUReady_flg"
  FrMCUReady/2 -> Terminator_18/1
  [BHAL_outputs] -> slr_VHAL_FrMCUReady4Pre_flg/1
  slr_VHAL_FrMCUReady4Pre_flg/1 -> FrMCUReady4Pre/1  "<VHAL_FrMCUReady4Pre_flg>"
  True_VHAL_FrMCUReady4Pre_flg/1 -> FrMCUReady4Pre/2
  [inp_CanValid_bus] -> slr1_19/1
  slr1_19/1 -> FrMCUReady4Pre/3  "<VINP_CANMsgValidMCUBF1_flg>"
  FrMCUReady4Pre/1 -> VINP_FrMCUReady4Pre_flg/1  "VINP_FrMCUReady4Pre_flg"
  FrMCUReady4Pre/2 -> Terminator_19/1
  [BHAL_outputs] -> slr_VHAL_FrMCUSysSta_enum/1
  slr_VHAL_FrMCUSysSta_enum/1 -> FrMCUSysSta/1  "<VHAL_FrMCUSysSta_enum>"
  True_VHAL_FrMCUSysSta_enum/1 -> FrMCUSysSta/2
  [inp_CanValid_bus] -> slr1_20/1
  slr1_20/1 -> FrMCUSysSta/3  "<VINP_CANMsgValidMCUBF1_flg>"
  FrMCUSysSta/1 -> VINP_FrMCUSysSta_enum/1  "VINP_FrMCUSysSta_enum"
  FrMCUSysSta/2 -> Terminator_20/1
  [BHAL_outputs] -> slr_VHAL_FrMCUTemp_C/1
  slr_VHAL_FrMCUTemp_C/1 -> FrMCUTemp/1  "<VHAL_FrMCUTemp_C>"
  True_VHAL_FrMCUTemp_C/1 -> FrMCUTemp/2
  [inp_CanValid_bus] -> slr1_21/1
  slr1_21/1 -> FrMCUTemp/3  "<VINP_CANMsgValidMCUBF1_flg>"
  FrMCUTemp/1 -> VINP_FrMCUTemp_C/1  "VINP_FrMCUTemp_C"
  FrMCUTemp/2 -> Terminator_21/1
  [BHAL_outputs] -> slr_VHAL_FrMotorAvailTq_Nm/1
  slr_VHAL_FrMotorAvailTq_Nm/1 -> FrMotorAvailTq/1  "<VHAL_FrMotorAvailTq_Nm>"
  True_VHAL_FrMotorAvailTq_Nm/1 -> FrMotorAvailTq/2
  [inp_CanValid_bus] -> slr1_22/1
  slr1_22/1 -> FrMotorAvailTq/3  "<VINP_CANMsgValidMCUBF1_flg>"
  FrMotorAvailTq/1 -> VINP_FrMotorAvailTq_Nm/1  "VINP_FrMotorAvailTq_Nm"
  FrMotorAvailTq/2 -> Terminator_22/1
  [BHAL_outputs] -> slr_VHAL_FrRegenAvailTq_Nm/1
  slr_VHAL_FrRegenAvailTq_Nm/1 -> FrRegenAvailTq/1  "<VHAL_FrRegenAvailTq_Nm>"
  True_VHAL_FrRegenAvailTq_Nm/1 -> FrRegenAvailTq/2
  [inp_CanValid_bus] -> slr1_23/1
  slr1_23/1 -> FrRegenAvailTq/3  "<VINP_CANMsgValidMCUBF1_flg>"
  FrRegenAvailTq/1 -> VINP_FrRegenAvailTq_Nm/1  "VINP_FrRegenAvailTq_Nm"
  FrRegenAvailTq/2 -> Terminator_23/1
  [BHAL_outputs] -> slr_VHAL_FrTMSpd_rpm/1
  slr_VHAL_FrTMSpd_rpm/1 -> FrTMSpd/1  "<VHAL_FrTMSpd_rpm>"
  True_VHAL_FrTMSpd_rpm/1 -> FrTMSpd/2
  [inp_CanValid_bus] -> slr1_24/1
  slr1_24/1 -> FrTMSpd/3  "<VINP_CANMsgValidMCUBF1_flg>"
  FrTMSpd/1 -> VINP_FrTMSpd_rpm/1  "VINP_FrTMSpd_rpm"
  FrTMSpd/2 -> Terminator_24/1
  [BHAL_outputs] -> slr_VHAL_FrTMTemp_C/1
  slr_VHAL_FrTMTemp_C/1 -> FrTMTemp/1  "<VHAL_FrTMTemp_C>"
  True_VHAL_FrTMTemp_C/1 -> FrTMTemp/2
  [inp_CanValid_bus] -> slr1_25/1
  slr1_25/1 -> FrTMTemp/3  "<VINP_CANMsgValidMCUBF1_flg>"
  FrTMTemp/1 -> VINP_FrTMTemp_C/1  "VINP_FrTMTemp_C"
  FrTMTemp/2 -> Terminator_25/1
  [BHAL_outputs] -> slr_VHAL_FrTMid_A/1
  slr_VHAL_FrTMid_A/1 -> FrTMid/1  "<VHAL_FrTMid_A>"
  True_VHAL_FrTMid_A/1 -> FrTMid/2
  [inp_CanValid_bus] -> slr1_26/1
  slr1_26/1 -> FrTMid/3  "<VINP_CANMsgValidMCUBF1_flg>"
  FrTMid/1 -> VINP_FrTMid_A/1  "VINP_FrTMid_A"
  FrTMid/2 -> Terminator_26/1
  [BHAL_outputs] -> slr_VHAL_FrTMiq_A/1
  slr_VHAL_FrTMiq_A/1 -> FrTMiq/1  "<VHAL_FrTMiq_A>"
  True_VHAL_FrTMiq_A/1 -> FrTMiq/2
  [inp_CanValid_bus] -> slr1_27/1
  slr1_27/1 -> FrTMiq/3  "<VINP_CANMsgValidMCUBF1_flg>"
  FrTMiq/1 -> VINP_FrTMiq_A/1  "VINP_FrTMiq_A"
  FrTMiq/2 -> Terminator_27/1
  [BHAL_outputs] -> slr_VHAL_MCUWarnF_enum/1
  slr_VHAL_MCUWarnF_enum/1 -> MCUWarnF/1  "<VHAL_MCUWarnF_enum>"
  True_VHAL_MCUWarnF_enum/1 -> MCUWarnF/2
  [inp_CanValid_bus] -> slr1_28/1
  slr1_28/1 -> MCUWarnF/3  "<VINP_CANMsgValidMCUBF1_flg>"
  MCUWarnF/1 -> VINP_MCUWarnF_enum/1  "VINP_MCUWarnF_enum"
  MCUWarnF/2 -> Terminator_28/1
  [BHAL_outputs] -> slr_VHAL_MCUBFRealPwrKwSta_kW/1
  slr_VHAL_MCUBFRealPwrKwSta_kW/1 -> MCUBFRealPwrKwSta/1  "<VHAL_MCUBFRealPwrKwSta_kW>"
  True_VHAL_MCUBFRealPwrKwSta_kW/1 -> MCUBFRealPwrKwSta/2
  [inp_CanValid_bus] -> slr1_29/1
  slr1_29/1 -> MCUBFRealPwrKwSta/3  "<VINP_CANMsgValidMCUBF1_flg>"
  MCUBFRealPwrKwSta/1 -> VINP_MCUBFRealPwrKwSta_kW/1  "VINP_MCUBFRealPwrKwSta_kW"
  MCUBFRealPwrKwSta/2 -> Terminator_29/1
